simulink model "Model_TranslationEngine64"  (R2022b)
settings: Solver=FixedStepDiscrete  StartTime=0.0  StopTime=5  RelTol=1e-3  EnableMultiTasking=on
InitFcn:
  | % Initialize model
  | ModelSettings=BTConfig.GetModelSettings();
  | 
  | ModelSettings.Validate();
  | 
  | ModelInit;
  | 
  | 
  | % load library data
  | GainLibrary_data;
  | % Load saved values from partition process
  | CapturedConstMask.LoadMapFromFile(bdroot)
StartFcn:
  | % make sure all the simulated RTC requests are found
  | %RTC_SIM_OBJ.ValidateREQs();
undefined symbols (not defined in the file or in its folder): AA, BPLP, Column, NumHFRefBPF, NumHFRefLPF, NumMusicChannels, Row, VolumeMuteConfig
libraries: TuneVar x925, TOP x490, FeaturePath x111, CapturedConstLib x52
(part 31 of 34)

== matlab function Model_TranslationEngine64/NEAR/Near1p1/DrProc/RouterDr/InnerLink/Trivial Translation ==
  data: OutMap output; Map input; nInRouterMask parameter
  events: trigger input FUNCTION_CALL_EVENT
function OutMap  = fcn(Map, nInRouterMask)
%#codegen

% ----- To access TuneVar maximum size, current size, and current value:
%   Note: TuneVar signals arrive with exposed variable size information.
%         The expressions below illustrate for the "Map" input argument.
%
%   size(Map.Value) : the maximum possible size of the Map variable
%
%   Tune.Size   : the current size of *valid* data in Map.Value
%
%   Map.Size(1) : Number of rows present in Map - this does not vary.
%
%   Map.Size(2) : Number of columns currently valid in Map - this is
%       the variable part of size that can change (if allowed by TuneVar).
%
%   Map.Value : the current value of the tune variable... but end-padded 
%       to the maximum available size with undefined/invalid data.
%
%   numel(Map.Value) : another way of looking at the maximum number of
%       elements that could arrive in Map.Value
%
% ----- To register an error, use the following method (works like printf):
%   TranslateError( <format string>, <arguments ... )
%   ... this error will cause the build process to abort.


% The below logic ensures that an output map gets filled in in the 
% "round robin" manner. This is to occur when the supplied map is shorter
% than the number of channel outputs. For instance,
% nChanIn = 4
% nChanOut = 9
% outputMapSupplied = [4 3 2 2]
% 
% This logic would run and return OutMap = [4 3 2 2 1 2 3 4 1]
%
% If no outputMap was supplied (i.e. = [];) THEN
% This logic would run and return OutMap = [1 2 3 4 1 2 3 4 1];


% First part finds the number of output map indices that were left blank
nChanOut = numel(Map.Value);
mapLength = Map.Size(2);
mapDifference = nChanOut - mapLength;
OutMap = int32(Map.Value);

% This loop appropriates the correct input channel number to the
% corresponding output channel, based on the mapDifference found above
if (mapLength == 1) && Map.Value(1) == 0
    mapLength = 0;
    mapDifference = nChanOut;
end
endOfMap = 0;
loopCount = 0;
while endOfMap < mapDifference
    for inputChan = 1 : nInRouterMask
        OutMap(mapLength+inputChan+loopCount) = inputChan;
        endOfMap = endOfMap + 1;
        if endOfMap == mapDifference
            break
        end
    end
    inputChan = 1;
    loopCount = loopCount + nInRouterMask;
end

== matlab function Model_TranslationEngine64/NEAR/Near1p1/DrProc/Upmixer1p1Dr/Subsystem1/Translation ==
  data: mix output single; F1 input; F2 input; F3 input; F4 input; F5 input; F6 input; F7 input; LFI0 input; LFT0 input; RFI0 input; RFT0 input; LSI0 input; LST0 input; RSI0 input; RST0 input; LCI0 input; LCT0 input; RCI0 input; RCT0 input; LFI1 input; LFT1 input; RFI1 input; RFT1 input; LSI1 input; LST1 input; RSI1 input; RST1 input; LCI1 input; LCT1 input; RCI1 input; RCT1 input; nv0l input; nv0r input; nv1l input; nv1r input; FrontPeripheralChannelCount parameter; HeadrestCount parameter; ChannelsPerHeadrest parameter
  events: trigger input FUNCTION_CALL_EVENT
function mix  = fcn(    F1,...
                        F2,...
                        F3,...
                        F4,...
                        F5,...
                        F6,...
                        F7,...
                        LFI0,...
                        LFT0,...
                        RFI0,...
                        RFT0,...
                        LSI0,...
                        LST0,...
                        RSI0,...
                        RST0,...
                        LCI0,...
                        LCT0,...
                        RCI0,...
                        RCT0,...
                        LFI1,...
                        LFT1,...
                        RFI1,...
                        RFT1,...
                        LSI1,...
                        LST1,...
                        RSI1,...
                        RST1,...
                        LCI1,...
                        LCT1,...
                        RCI1,...
                        RCT1,...
                        nv0l,...
                        nv0r,...
                        nv1l,...
                        nv1r, ...
                        FrontPeripheralChannelCount, HeadrestCount, ChannelsPerHeadrest)

% mix = cat(3, F1.Value, F1.Value);                    
% mix = cat(              3,... 
%                         F1.Value,...
%                         F2.Value,...
%                         F3.Value,...
%                         F4.Value,...
%                         F5.Value,...
%                         F6.Value,...
%                         F7.Value,...
%                         LFI0.Value,...
%                         LFT0.Value,...
%                         RFI0.Value,...
%                         RFT0.Value,...
%                         LSI0.Value,...
%                         LST0.Value,...
%                         RSI0.Value,...
%                         RST0.Value,...
%                         LCI0.Value,...
%                         LCT0.Value,...
%                         RCI0.Value,...
%                         RCT0.Value,...
%                         LFI1.Value,...
%                         LFT1.Value,...
%                         RFI1.Value,...
%                         RFT1.Value,...
%                         LSI1.Value,...
%                         LST1.Value,...
%                         RSI1.Value,...
%                         RST1.Value,...
%                         LCI1.Value,...
%                         LCT1.Value,...
%                         RCI1.Value,...
%                         RCT1.Value,...
%                         nv0l.Value,...
%                         nv0r.Value,...
%                         nv1l.Value,...
%                         nv1r.Value);

% f = size(fArr, 1);
% hr = size(hrArr, 1);
% cph = size(cphArr, 1);
f = FrontPeripheralChannelCount;
hr = HeadrestCount;
cph = ChannelsPerHeadrest;
mixSize = f + hr*cph;
% s = size(F1.Value, 1);
s = size(LFI0.Value, 1);
mix = single(zeros(s, s, mixSize));

x = cat(3, F1.Value, F2.Value, F3.Value, F4.Value, F5.Value, F6.Value, F7.Value);
mix(:,:,1:f) = x(:,:,1:f);
if cph == 14
    x = cat(        3,... 
                    LFI0.Value,...
                    LFT0.Value,...
                    RFI0.Value,...
                    RFT0.Value,...
                    LSI0.Value,...
                    LST0.Value,...
                    RSI0.Value,...
                    RST0.Value,...
                    LCI0.Value,...
                    LCT0.Value,...
                    RCI0.Value,...
                    RCT0.Value);
    mix(:,:,f+1:f+12) = x;
	if hr == 2
        x = cat(    3,... 
                    LFI1.Value,...
                    LFT1.Value,...
                    RFI1.Value,...
                    RFT1.Value,...
                    LSI1.Value,...
                    LST1.Value,...
                    RSI1.Value,...
                    RST1.Value,...
                    LCI1.Value,...
                    LCT1.Value,...
                    RCI1.Value,...
                    RCT1.Value);
        mix(:,:,f+13:f+24) = x;
	end
end
x = cat(    3,... 
            nv0l.Value,...
            nv0r.Value);
mix(:,:,f+((cph-2)*hr)+1:f+((cph-2)*hr)+2) = x;
if hr == 2
	x = cat(    3,... 
                nv1l.Value,...
                nv1r.Value);
    mix(:,:,f+((cph-2)*hr)+3:f+((cph-2)*hr)+4) = x;
end
end

== matlab function Model_TranslationEngine64/NEAR/Near1p1/FrProc/Subsystem/FsEQFr/Pooliir/PoolIirTunableWithReset/Translation ==
  data: RawSOS input; NumStages input; PoolNumStages output; PoolCoeffs output; MaxNumStages parameter; VariantUint8 parameter; NumChannels input
  events: trigger input FUNCTION_CALL_EVENT
function [PoolNumStages, PoolCoeffs] = pooliirTranslation(RawSOS, NumStages, MaxNumStages, VariantUint8,  NumChannels)
%#codegen

% Translation from raw SOS for pool SOS

% Some build time sanity size checking before calling the translation
if numel(NumStages.Value) ~= NumChannels
    error('Size of num stages has to match number of input channels')
end

if RawSOS.Size(2) ~= 6
    error ('Coefficient pool matrix must have 6 columns')
end

[PoolNumStages, PoolCoeffs] = poolIirTranslation(RawSOS, NumStages, MaxNumStages, VariantUint8);

% VariantStr = char(VariantUint8);
% switch (VariantStr)
%     case {"Generic","SharcPlusCore"}
%         % These variants order biquad coefficients in a compacted form
%         [PoolNumStages, PoolCoeffs] = pooliirTranslationFcn(RawSOS, NumStages, MaxNumStages);
%     case {"SharcPlusAccelGul","SharcPlusAccelGxp"}
%         % These variants order biquad coefficients for the ADI accelerator
%         [PoolNumStages, PoolCoeffs] = pooliirAccelTranslationFcn(RawSOS, NumStages, MaxNumStages);
%     case{"Hexagon"}
%         % Hexagon specific order for biquad coefficients 
%         [PoolNumStages, PoolCoeffs] = PoolIirHexagonTranslationFcn(RawSOS, NumStages, MaxNumStages);
%     case{"ArmNeonV7V8"}
%         [PoolNumStages, PoolCoeffs] = PoolIirArmNeonV7V8TranslationFcn(RawSOS, NumStages, MaxNumStages);
%     otherwise
%         % This is a build-time error, not a translation error. The
%         % selected build-time variant is not supported for translation
%         error('Invalid implementation type: [%s]', VariantStr);
% end

end

== matlab function Model_TranslationEngine64/NEAR/Near1p1/FrProc/Subsystem/HrEQFr/Subsystem2/Translation ==
  data: eqdelays output single; driversrc1 input; driversrc2 input; driversrc3 input; driversrc4 input; passengersrc1 input; passengersrc2 input; passengersrc3 input; passengersrc4 input; NumHeadrestSpeakers parameter; AnnChannelCount parameter
  events: trigger input FUNCTION_CALL_EVENT
function eqdelays  = fcn(driversrc1, driversrc2, driversrc3, driversrc4, passengersrc1, passengersrc2, passengersrc3, passengersrc4, NumHeadrestSpeakers, AnnChannelCount)
    switch NumHeadrestSpeakers
        case 1
            switch AnnChannelCount
                case 1
                    eqdelays = single([driversrc1.Value, driversrc2.Value]);
                case 2
                    eqdelays = single([driversrc1.Value, driversrc2.Value]);
                case 3
                    eqdelays = single([driversrc1.Value, driversrc2.Value, driversrc3.Value]);
                case 4
                    eqdelays = single([driversrc1.Value, driversrc2.Value, driversrc3.Value, driversrc4.Value]);
            end
        case 2
            switch AnnChannelCount
                case 1
                    eqdelays = single([driversrc1.Value, driversrc2.Value, passengersrc1.Value, passengersrc2.Value]);
                case 2
                    eqdelays = single([driversrc1.Value, driversrc2.Value, passengersrc1.Value, passengersrc2.Value]);
                case 3
                    eqdelays = single([driversrc1.Value, driversrc2.Value, driversrc3.Value, passengersrc1.Value, passengersrc2.Value, passengersrc3.Value]);
                case 4
                    eqdelays = single([driversrc1.Value, driversrc2.Value, driversrc3.Value, driversrc4.Value, passengersrc1.Value, passengersrc2.Value, passengersrc3.Value, passengersrc4.Value]);
            end
    end

end

== matlab function Model_TranslationEngine64/NEAR/Near1p1/FrProc/Subsystem/HrEQFr/PoolIirTunable/PoolIirTunableWithReset/Translation ==
  data: RawSOS input; NumStages input; PoolNumStages output; PoolCoeffs output; MaxNumStages parameter; VariantUint8 parameter; NumChannels input
  events: trigger input FUNCTION_CALL_EVENT
function [PoolNumStages, PoolCoeffs] = pooliirTranslation(RawSOS, NumStages, MaxNumStages, VariantUint8,  NumChannels)
%#codegen

% Translation from raw SOS for pool SOS

% Some build time sanity size checking before calling the translation
if numel(NumStages.Value) ~= NumChannels
    error('Size of num stages has to match number of input channels')
end

if RawSOS.Size(2) ~= 6
    error ('Coefficient pool matrix must have 6 columns')
end

[PoolNumStages, PoolCoeffs] = poolIirTranslation(RawSOS, NumStages, MaxNumStages, VariantUint8);

% VariantStr = char(VariantUint8);
% switch (VariantStr)
%     case {"Generic","SharcPlusCore"}
%         % These variants order biquad coefficients in a compacted form
%         [PoolNumStages, PoolCoeffs] = pooliirTranslationFcn(RawSOS, NumStages, MaxNumStages);
%     case {"SharcPlusAccelGul","SharcPlusAccelGxp"}
%         % These variants order biquad coefficients for the ADI accelerator
%         [PoolNumStages, PoolCoeffs] = pooliirAccelTranslationFcn(RawSOS, NumStages, MaxNumStages);
%     case{"Hexagon"}
%         % Hexagon specific order for biquad coefficients 
%         [PoolNumStages, PoolCoeffs] = PoolIirHexagonTranslationFcn(RawSOS, NumStages, MaxNumStages);
%     case{"ArmNeonV7V8"}
%         [PoolNumStages, PoolCoeffs] = PoolIirArmNeonV7V8TranslationFcn(RawSOS, NumStages, MaxNumStages);
%     otherwise
%         % This is a build-time error, not a translation error. The
%         % selected build-time variant is not supported for translation
%         error('Invalid implementation type: [%s]', VariantStr);
% end

end

== matlab function Model_TranslationEngine64/NEAR/Near1p1/VolumeMute/AnnouncementLevelDetector/ch2_level/hold_time/sec2samples ==
  data: y output; u input; FrameRate parameter
  events: trigger input FUNCTION_CALL_EVENT
function y  = fcn(u,FrameRate)
%#codegen

y = ceil(u.Value*FrameRate);

== matlab function Model_TranslationEngine64/ModelPreAmp/DecRate/AudioPilot35/Audiopilot_3_5/GainApplication/Compensation/MidrangeLpf/LinkwitzRiley ==
  data: num output; freq input; denom output; SampleRate parameter
  events: trigger input FUNCTION_CALL_EVENT
function [num,denom] = fcn(freq,SampleRate)
% Forms the numerator and denominator coefficients
% for a 4th order Linkwitz-Riley low-pass filter with 
% the specified cutoff frequency 
%#codegen

Fc = freq.Value;
FiltOrder = 4;  % This is hard-coded

[Z,P,K] = LinkwitzRileyFiltDesign(FiltOrder,Fc/(SampleRate/2),'low');
[num, denom] = zp2tf(Z,P,K);

== matlab function Model_TranslationEngine64/NEAR/Near1p1/FrProc/Subsystem/RouterFr/InnerLink/Trivial Translation ==
  data: OutMap output; Map input; nInRouterMask parameter
  events: trigger input FUNCTION_CALL_EVENT
function OutMap  = fcn(Map, nInRouterMask)
%#codegen

% ----- To access TuneVar maximum size, current size, and current value:
%   Note: TuneVar signals arrive with exposed variable size information.
%         The expressions below illustrate for the "Map" input argument.
%
%   size(Map.Value) : the maximum possible size of the Map variable
%
%   Tune.Size   : the current size of *valid* data in Map.Value
%
%   Map.Size(1) : Number of rows present in Map - this does not vary.
%
%   Map.Size(2) : Number of columns currently valid in Map - this is
%       the variable part of size that can change (if allowed by TuneVar).
%
%   Map.Value : the current value of the tune variable... but end-padded 
%       to the maximum available size with undefined/invalid data.
%
%   numel(Map.Value) : another way of looking at the maximum number of
%       elements that could arrive in Map.Value
%
% ----- To register an error, use the following method (works like printf):
%   TranslateError( <format string>, <arguments ... )
%   ... this error will cause the build process to abort.


% The below logic ensures that an output map gets filled in in the 
% "round robin" manner. This is to occur when the supplied map is shorter
% than the number of channel outputs. For instance,
% nChanIn = 4
% nChanOut = 9
% outputMapSupplied = [4 3 2 2]
% 
% This logic would run and return OutMap = [4 3 2 2 1 2 3 4 1]
%
% If no outputMap was supplied (i.e. = [];) THEN
% This logic would run and return OutMap = [1 2 3 4 1 2 3 4 1];


% First part finds the number of output map indices that were left blank
nChanOut = numel(Map.Value);
mapLength = Map.Size(2);
mapDifference = nChanOut - mapLength;
OutMap = int32(Map.Value);

% This loop appropriates the correct input channel number to the
% corresponding output channel, based on the mapDifference found above
if (mapLength == 1) && Map.Value(1) == 0
    mapLength = 0;
    mapDifference = nChanOut;
end
endOfMap = 0;
loopCount = 0;
while endOfMap < mapDifference
    for inputChan = 1 : nInRouterMask
        OutMap(mapLength+inputChan+loopCount) = inputChan;
        endOfMap = endOfMap + 1;
        if endOfMap == mapDifference
            break
        end
    end
    inputChan = 1;
    loopCount = loopCount + nInRouterMask;
end

== matlab function Model_TranslationEngine64/NEAR/Near1p1/FrProc/Subsystem/Upmixer1p1Fr/Subsystem1/Translation ==
  data: mix output single; F1 input; F2 input; F3 input; F4 input; F5 input; F6 input; F7 input; LFI0 input; LFT0 input; RFI0 input; RFT0 input; LSI0 input; LST0 input; RSI0 input; RST0 input; LCI0 input; LCT0 input; RCI0 input; RCT0 input; LFI1 input; LFT1 input; RFI1 input; RFT1 input; LSI1 input; LST1 input; RSI1 input; RST1 input; LCI1 input; LCT1 input; RCI1 input; RCT1 input; nv0l input; nv0r input; nv1l input; nv1r input; FrontPeripheralChannelCount parameter; HeadrestCount parameter; ChannelsPerHeadrest parameter
  events: trigger input FUNCTION_CALL_EVENT
function mix  = fcn(    F1,...
                        F2,...
                        F3,...
                        F4,...
                        F5,...
                        F6,...
                        F7,...
                        LFI0,...
                        LFT0,...
                        RFI0,...
                        RFT0,...
                        LSI0,...
                        LST0,...
                        RSI0,...
                        RST0,...
                        LCI0,...
                        LCT0,...
                        RCI0,...
                        RCT0,...
                        LFI1,...
                        LFT1,...
                        RFI1,...
                        RFT1,...
                        LSI1,...
                        LST1,...
                        RSI1,...
                        RST1,...
                        LCI1,...
                        LCT1,...
                        RCI1,...
                        RCT1,...
                        nv0l,...
                        nv0r,...
                        nv1l,...
                        nv1r, ...
                        FrontPeripheralChannelCount, HeadrestCount, ChannelsPerHeadrest)

% mix = cat(3, F1.Value, F1.Value);                    
% mix = cat(              3,... 
%                         F1.Value,...
%                         F2.Value,...
%                         F3.Value,...
%                         F4.Value,...
%                         F5.Value,...
%                         F6.Value,...
%                         F7.Value,...
%                         LFI0.Value,...
%                         LFT0.Value,...
%                         RFI0.Value,...
%                         RFT0.Value,...
%                         LSI0.Value,...
%                         LST0.Value,...
%                         RSI0.Value,...
%                         RST0.Value,...
%                         LCI0.Value,...
%                         LCT0.Value,...
%                         RCI0.Value,...
%                         RCT0.Value,...
%                         LFI1.Value,...
%                         LFT1.Value,...
%                         RFI1.Value,...
%                         RFT1.Value,...
%                         LSI1.Value,...
%                         LST1.Value,...
%                         RSI1.Value,...
%                         RST1.Value,...
%                         LCI1.Value,...
%                         LCT1.Value,...
%                         RCI1.Value,...
%                         RCT1.Value,...
%                         nv0l.Value,...
%                         nv0r.Value,...
%                         nv1l.Value,...
%                         nv1r.Value);

% f = size(fArr, 1);
% hr = size(hrArr, 1);
% cph = size(cphArr, 1);
f = FrontPeripheralChannelCount;
hr = HeadrestCount;
cph = ChannelsPerHeadrest;
mixSize = f + hr*cph;
% s = size(F1.Value, 1);
s = size(LFI0.Value, 1);
mix = single(zeros(s, s, mixSize));

x = cat(3, F1.Value, F2.Value, F3.Value, F4.Value, F5.Value, F6.Value, F7.Value);
mix(:,:,1:f) = x(:,:,1:f);
if cph == 14
    x = cat(        3,... 
                    LFI0.Value,...
                    LFT0.Value,...
                    RFI0.Value,...
                    RFT0.Value,...
                    LSI0.Value,...
                    LST0.Value,...
                    RSI0.Value,...
                    RST0.Value,...
                    LCI0.Value,...
                    LCT0.Value,...
                    RCI0.Value,...
                    RCT0.Value);
    mix(:,:,f+1:f+12) = x;
	if hr == 2
        x = cat(    3,... 
                    LFI1.Value,...
                    LFT1.Value,...
                    RFI1.Value,...
                    RFT1.Value,...
                    LSI1.Value,...
                    LST1.Value,...
                    RSI1.Value,...
                    RST1.Value,...
                    LCI1.Value,...
                    LCT1.Value,...
                    RCI1.Value,...
                    RCT1.Value);
        mix(:,:,f+13:f+24) = x;
	end
end
x = cat(    3,... 
            nv0l.Value,...
            nv0r.Value);
mix(:,:,f+((cph-2)*hr)+1:f+((cph-2)*hr)+2) = x;
if hr == 2
	x = cat(    3,... 
                nv1l.Value,...
                nv1r.Value);
    mix(:,:,f+((cph-2)*hr)+3:f+((cph-2)*hr)+4) = x;
end
end

== matlab function Model_TranslationEngine64/NEAR/Near1p1/VolumeMute/AnnouncementLevelDetector/ch2_level/slow_decay/sec2samples ==
  data: y output; u input; FrameRate parameter
  events: trigger input FUNCTION_CALL_EVENT
function y  = fcn(u,FrameRate)
%#codegen

y = -abs(u.Value/FrameRate);

== matlab function Model_TranslationEngine64/NEAR/Near1p1/VolumeMute/AnnouncementLevelDetector/ch3_level/fast_decay/sec2samples ==
  data: y output; u input; FrameRate parameter
  events: trigger input FUNCTION_CALL_EVENT
function y  = fcn(u,FrameRate)
%#codegen

y = -abs(u.Value/FrameRate);

== matlab function Model_TranslationEngine64/NEAR/Near1p1/VolumeMute/AnnouncementLevelDetector/ch3_level/hold_margin/SetPositive ==
  data: TOP output single; Tune input
  events: trigger input FUNCTION_CALL_EVENT
function TOP = fcn(Tune)
%#codegen

TOP = abs(Tune.Value);

== matlab function Model_TranslationEngine64/NEAR/Near1p1/VolumeMute/AnnouncementLevelDetector/ch3_level/hold_time/sec2samples ==
  data: y output; u input; FrameRate parameter
  events: trigger input FUNCTION_CALL_EVENT
function y  = fcn(u,FrameRate)
%#codegen

y = ceil(u.Value*FrameRate);

== matlab function Model_TranslationEngine64/NEAR/Near1p1/VolumeMute/AnnouncementLevelDetector/ch3_level/slow_decay/sec2samples ==
  data: y output; u input; FrameRate parameter
  events: trigger input FUNCTION_CALL_EVENT
function y  = fcn(u,FrameRate)
%#codegen

y = -abs(u.Value/FrameRate);

== matlab function Model_TranslationEngine64/ModelPreAmp/DecRate/AudioPilot35/Audiopilot_3_5/NoiseEstimationVariant/RegularNoiseEstimation/HFNoiseEstimatorCoh/PreProcessing/Anti-Aliasing Filter/InnerLink/PoolIirTunableWithReset/Translation ==
  data: RawSOS input; NumStages input; PoolNumStages output; PoolCoeffs output; MaxNumStages parameter; VariantUint8 parameter; NumChannels input
  events: trigger input FUNCTION_CALL_EVENT
function [PoolNumStages, PoolCoeffs] = pooliirTranslation(RawSOS, NumStages, MaxNumStages, VariantUint8,  NumChannels)
%#codegen

% Translation from raw SOS for pool SOS

% Some build time sanity size checking before calling the translation
if numel(NumStages.Value) ~= NumChannels
    error('Size of num stages has to match number of input channels')
end

if RawSOS.Size(2) ~= 6
    error ('Coefficient pool matrix must have 6 columns')
end

[PoolNumStages, PoolCoeffs] = poolIirTranslation(RawSOS, NumStages, MaxNumStages, VariantUint8);

% VariantStr = char(VariantUint8);
% switch (VariantStr)
%     case {"Generic","SharcPlusCore"}
%         % These variants order biquad coefficients in a compacted form
%         [PoolNumStages, PoolCoeffs] = pooliirTranslationFcn(RawSOS, NumStages, MaxNumStages);
%     case {"SharcPlusAccelGul","SharcPlusAccelGxp"}
%         % These variants order biquad coefficients for the ADI accelerator
%         [PoolNumStages, PoolCoeffs] = pooliirAccelTranslationFcn(RawSOS, NumStages, MaxNumStages);
%     case{"Hexagon"}
%         % Hexagon specific order for biquad coefficients 
%         [PoolNumStages, PoolCoeffs] = PoolIirHexagonTranslationFcn(RawSOS, NumStages, MaxNumStages);
%     case{"ArmNeonV7V8"}
%         [PoolNumStages, PoolCoeffs] = PoolIirArmNeonV7V8TranslationFcn(RawSOS, NumStages, MaxNumStages);
%     otherwise
%         % This is a build-time error, not a translation error. The
%         % selected build-time variant is not supported for translation
%         error('Invalid implementation type: [%s]', VariantStr);
% end

end

== matlab function Model_TranslationEngine64/NEAR/Near1p1/VolumeMute/AnnouncementLevelDetector/ch4_level/fast_decay/sec2samples ==
  data: y output; u input; FrameRate parameter
  events: trigger input FUNCTION_CALL_EVENT
function y  = fcn(u,FrameRate)
%#codegen

y = -abs(u.Value/FrameRate);

== matlab function Model_TranslationEngine64/NEAR/Near1p1/VolumeMute/AnnouncementLevelDetector/ch4_level/hold_margin/SetPositive ==
  data: TOP output single; Tune input
  events: trigger input FUNCTION_CALL_EVENT
function TOP = fcn(Tune)
%#codegen

TOP = abs(Tune.Value);

== matlab function Model_TranslationEngine64/NEAR/Near1p1/VolumeMute/AnnouncementLevelDetector/ch4_level/hold_time/sec2samples ==
  data: y output; u input; FrameRate parameter
  events: trigger input FUNCTION_CALL_EVENT
function y  = fcn(u,FrameRate)
%#codegen

y = ceil(u.Value*FrameRate);

== matlab function Model_TranslationEngine64/NEAR/Near1p1/VolumeMute/AnnouncementLevelDetector/ch4_level/slow_decay/sec2samples ==
  data: y output; u input; FrameRate parameter
  events: trigger input FUNCTION_CALL_EVENT
function y  = fcn(u,FrameRate)
%#codegen

y = -abs(u.Value/FrameRate);

== matlab function Model_TranslationEngine64/NEAR/Near1p1/VolumeMute/VolMuteCh1/Ann1NonEntGainCalc/TuneTOP8/translation ==
  data: Num output size=[1,2]; tau input size=1; Den output size=[1,2]; Fd parameter
  events: trigger input FUNCTION_CALL_EVENT
function [Num, Den]  = fcn(tau, Fd)
%
% Calculate coefficients for single pole LPF
%

Wc      = 1/(tau.Value*Fd);
sinCoef = sin(Wc);
cosCoef = cos(Wc);
coef    = (1-sinCoef)/cosCoef;

Num = double([1-coef 0]);
Den =  double([1 -(coef)]);

== matlab function Model_TranslationEngine64/NEAR/Near1p1/VolumeMute/AnnouncementLevelDetector/PreProcessing/PreEmphasisShelfFilter/PoolIirTunableWithReset/Translation ==
  data: RawSOS input; NumStages input; PoolNumStages output; PoolCoeffs output; MaxNumStages parameter; VariantUint8 parameter; NumChannels input
  events: trigger input FUNCTION_CALL_EVENT
function [PoolNumStages, PoolCoeffs] = pooliirTranslation(RawSOS, NumStages, MaxNumStages, VariantUint8,  NumChannels)
%#codegen

% Translation from raw SOS for pool SOS

% Some build time sanity size checking before calling the translation
if numel(NumStages.Value) ~= NumChannels
    error('Size of num stages has to match number of input channels')
end

if RawSOS.Size(2) ~= 6
    error ('Coefficient pool matrix must have 6 columns')
end

[PoolNumStages, PoolCoeffs] = poolIirTranslation(RawSOS, NumStages, MaxNumStages, VariantUint8);

% VariantStr = char(VariantUint8);
% switch (VariantStr)
%     case {"Generic","SharcPlusCore"}
%         % These variants order biquad coefficients in a compacted form
%         [PoolNumStages, PoolCoeffs] = pooliirTranslationFcn(RawSOS, NumStages, MaxNumStages);
%     case {"SharcPlusAccelGul","SharcPlusAccelGxp"}
%         % These variants order biquad coefficients for the ADI accelerator
%         [PoolNumStages, PoolCoeffs] = pooliirAccelTranslationFcn(RawSOS, NumStages, MaxNumStages);
%     case{"Hexagon"}
%         % Hexagon specific order for biquad coefficients 
%         [PoolNumStages, PoolCoeffs] = PoolIirHexagonTranslationFcn(RawSOS, NumStages, MaxNumStages);
%     case{"ArmNeonV7V8"}
%         [PoolNumStages, PoolCoeffs] = PoolIirArmNeonV7V8TranslationFcn(RawSOS, NumStages, MaxNumStages);
%     otherwise
%         % This is a build-time error, not a translation error. The
%         % selected build-time variant is not supported for translation
%         error('Invalid implementation type: [%s]', VariantStr);
% end

end

== matlab function Model_TranslationEngine64/NEAR/Near1p1/VolumeMute/VolMuteCh2/Ann2NonEntVncApplied/nonentVNCApplied_subsystem/TuneTOP/Translation ==
  data: Num output; tau input; Fs input; L input; Den output
  events: trigger input FUNCTION_CALL_EVENT
function [Num, Den]  = fcn(tau, Fs, L)

f0 = 1/tau.Value;   % Approximation of cutoff freq from lpf filter time constant

fs_lpf = Fs/L;        % lpf filtter sample rate

% [Num, Den]= butter(1,2*f0/fs_lpf);  % butter() doesn't work with dynamic parameters
[Num, Den] = firstOrderButter(fs_lpf,f0);  % Calculation of lpf filter coefficients

== matlab function Model_TranslationEngine64/NEAR/Near1p1/VolumeMute/VolMuteCh2/Ann2NonEntGainCalc/TuneTOP8/translation ==
  data: Num output size=[1,2]; tau input size=1; Den output size=[1,2]; Fd parameter
  events: trigger input FUNCTION_CALL_EVENT
function [Num, Den]  = fcn(tau, Fd)
%
% Calculate coefficients for single pole LPF
%

Wc      = 1/(tau.Value*Fd);
sinCoef = sin(Wc);
cosCoef = cos(Wc);
coef    = (1-sinCoef)/cosCoef;

Num = double([1-coef 0]);
Den =  double([1 -(coef)]);

== matlab function Model_TranslationEngine64/NEAR/Near1p1/VolumeMute/VolMuteCh3/Ann3NonEntVncApplied/nonentVNCApplied_subsystem/TuneTOP/Translation ==
  data: Num output; tau input; Fs input; L input; Den output
  events: trigger input FUNCTION_CALL_EVENT
function [Num, Den]  = fcn(tau, Fs, L)

f0 = 1/tau.Value;   % Approximation of cutoff freq from lpf filter time constant

fs_lpf = Fs/L;        % lpf filtter sample rate

% [Num, Den]= butter(1,2*f0/fs_lpf);  % butter() doesn't work with dynamic parameters
[Num, Den] = firstOrderButter(fs_lpf,f0);  % Calculation of lpf filter coefficients

== matlab function Model_TranslationEngine64/NEAR/Near1p1/VolumeMute/VolMuteCh3/Ann3NonEntGainCalc/TuneTOP8/translation ==
  data: Num output size=[1,2]; tau input size=1; Den output size=[1,2]; Fd parameter
  events: trigger input FUNCTION_CALL_EVENT
function [Num, Den]  = fcn(tau, Fd)
%
% Calculate coefficients for single pole LPF
%

Wc      = 1/(tau.Value*Fd);
sinCoef = sin(Wc);
cosCoef = cos(Wc);
coef    = (1-sinCoef)/cosCoef;

Num = double([1-coef 0]);
Den =  double([1 -(coef)]);

== matlab function Model_TranslationEngine64/NEAR/Near1p1/VolumeMute/VolMuteCh4/Ann4NonEntVncApplied/nonentVNCApplied_subsystem/TuneTOP/Translation ==
  data: Num output; tau input; Fs input; L input; Den output
  events: trigger input FUNCTION_CALL_EVENT
function [Num, Den]  = fcn(tau, Fs, L)

f0 = 1/tau.Value;   % Approximation of cutoff freq from lpf filter time constant

fs_lpf = Fs/L;        % lpf filtter sample rate

% [Num, Den]= butter(1,2*f0/fs_lpf);  % butter() doesn't work with dynamic parameters
[Num, Den] = firstOrderButter(fs_lpf,f0);  % Calculation of lpf filter coefficients

== matlab function Model_TranslationEngine64/NEAR/Near1p1/VolumeMute/VolMuteCh1/Volume/volume table translation ==
  data: Table_Idx output; Table_dB output; VolumeTable input
  events: trigger input FUNCTION_CALL_EVENT
function [Table_Idx,Table_dB] = fcn(VolumeTable)
%#codegen
%
% Demux Volume Table matrix into an index vector amd gain vector
%

% Set up the size and datatype of our TOP outputs:
maxTableSize = numel(VolumeTable.Value) / 2;
idxType = 'uint8';
idxStorageType = 'uint32';
dbType = 'single';
Table_Idx = zeros(1,maxTableSize,idxStorageType);
Table_dB = zeros(1,maxTableSize,dbType);

% separate the pairs into their index and value components
givenPairs = VolumeTable.Size(1);
indexes = VolumeTable.Value(1:givenPairs,1);
values = VolumeTable.Value(1:givenPairs,2);

% then sort and ignore duplicates
[cleanIdx,map] = unique(indexes);

% Validate input sizes
numPairs = numel(map);
argName='VolumeTable';

% Validate: enough data?
if (numPairs < 2)
    TranslateError('%s must have at least 2 index pairs. Encounted value with only %f pairs\n', argName, numPairs);
end

% Validate: Highest index still below 1.0?
if (cleanIdx(end) > 1)
    TranslateError('%s out of range table index %f encountered. Index must be between 0 and 1.\n',argName,cleanIdx(end));
end

% fill in the table buffer with provided pairs
for i=1:numPairs
    Table_Idx(i) = intmax(idxType) * cleanIdx(i);
    Table_dB(i) = values(map(i));
end
% fill the rest of the table buffer with the last entry
for j=numel(map)+1:maxTableSize
    Table_Idx(j) = Table_Idx(numPairs);
    Table_dB(j) =  Table_dB(numPairs);
end

end

== matlab function Model_TranslationEngine64/NEAR/Near1p1/VolumeMute/VolMuteCh4/Ann4NonEntGainCalc/TuneTOP8/translation ==
  data: Num output size=[1,2]; tau input size=1; Den output size=[1,2]; Fd parameter
  events: trigger input FUNCTION_CALL_EVENT
function [Num, Den]  = fcn(tau, Fd)
%
% Calculate coefficients for single pole LPF
%

Wc      = 1/(tau.Value*Fd);
sinCoef = sin(Wc);
cosCoef = cos(Wc);
coef    = (1-sinCoef)/cosCoef;

Num = double([1-coef 0]);
Den =  double([1 -(coef)]);

== matlab function Model_TranslationEngine64/ModelPreAmp/DecRate/AudioPilot35/Audiopilot_3_5/GainCalculation/BoostMapAdjustment/AudiopilotOn/Bass0Enable ==
  data: on input; slopeOut output; slope input
  events: trigger input FUNCTION_CALL_EVENT
function slopeOut  = enable(on,slope)
%#codegen
slopeOut = slope.Value * on.Value;

== matlab function Model_TranslationEngine64/PostProcess/PostProcess/PostLimiterEQ/PoolIirTunableWithReset/Translation ==
  data: RawSOS input; NumStages input; PoolNumStages output; PoolCoeffs output; MaxNumStages parameter; VariantUint8 parameter; NumChannels input
  events: trigger input FUNCTION_CALL_EVENT
function [PoolNumStages, PoolCoeffs] = pooliirTranslation(RawSOS, NumStages, MaxNumStages, VariantUint8,  NumChannels)
%#codegen

% Translation from raw SOS for pool SOS

% Some build time sanity size checking before calling the translation
if numel(NumStages.Value) ~= NumChannels
    error('Size of num stages has to match number of input channels')
end

if RawSOS.Size(2) ~= 6
    error ('Coefficient pool matrix must have 6 columns')
end

[PoolNumStages, PoolCoeffs] = poolIirTranslation(RawSOS, NumStages, MaxNumStages, VariantUint8);

% VariantStr = char(VariantUint8);
% switch (VariantStr)
%     case {"Generic","SharcPlusCore"}
%         % These variants order biquad coefficients in a compacted form
%         [PoolNumStages, PoolCoeffs] = pooliirTranslationFcn(RawSOS, NumStages, MaxNumStages);
%     case {"SharcPlusAccelGul","SharcPlusAccelGxp"}
%         % These variants order biquad coefficients for the ADI accelerator
%         [PoolNumStages, PoolCoeffs] = pooliirAccelTranslationFcn(RawSOS, NumStages, MaxNumStages);
%     case{"Hexagon"}
%         % Hexagon specific order for biquad coefficients 
%         [PoolNumStages, PoolCoeffs] = PoolIirHexagonTranslationFcn(RawSOS, NumStages, MaxNumStages);
%     case{"ArmNeonV7V8"}
%         [PoolNumStages, PoolCoeffs] = PoolIirArmNeonV7V8TranslationFcn(RawSOS, NumStages, MaxNumStages);
%     otherwise
%         % This is a build-time error, not a translation error. The
%         % selected build-time variant is not supported for translation
%         error('Invalid implementation type: [%s]', VariantStr);
% end

end

== matlab function Model_TranslationEngine64/NEAR/Near1p1/VolumeMute/VolMuteCh2/Volume/volume table translation ==
  data: Table_Idx output; Table_dB output; VolumeTable input
  events: trigger input FUNCTION_CALL_EVENT
function [Table_Idx,Table_dB] = fcn(VolumeTable)
%#codegen
%
% Demux Volume Table matrix into an index vector amd gain vector
%

% Set up the size and datatype of our TOP outputs:
maxTableSize = numel(VolumeTable.Value) / 2;
idxType = 'uint8';
idxStorageType = 'uint32';
dbType = 'single';
Table_Idx = zeros(1,maxTableSize,idxStorageType);
Table_dB = zeros(1,maxTableSize,dbType);

% separate the pairs into their index and value components
givenPairs = VolumeTable.Size(1);
indexes = VolumeTable.Value(1:givenPairs,1);
values = VolumeTable.Value(1:givenPairs,2);

% then sort and ignore duplicates
[cleanIdx,map] = unique(indexes);

% Validate input sizes
numPairs = numel(map);
argName='VolumeTable';

% Validate: enough data?
if (numPairs < 2)
    TranslateError('%s must have at least 2 index pairs. Encounted value with only %f pairs\n', argName, numPairs);
end

% Validate: Highest index still below 1.0?
if (cleanIdx(end) > 1)
    TranslateError('%s out of range table index %f encountered. Index must be between 0 and 1.\n',argName,cleanIdx(end));
end

% fill in the table buffer with provided pairs
for i=1:numPairs
    Table_Idx(i) = intmax(idxType) * cleanIdx(i);
    Table_dB(i) = values(map(i));
end
% fill the rest of the table buffer with the last entry
for j=numel(map)+1:maxTableSize
    Table_Idx(j) = Table_Idx(numPairs);
    Table_dB(j) =  Table_dB(numPairs);
end

end

== matlab function Model_TranslationEngine64/PostProcess/PostProcess/Limiter/Limiter/MATLAB Function1 ==
  data: u input; y output; Fs input
  events: trigger input FUNCTION_CALL_EVENT
function y = fcn(u, Fs)

% Convert from dB to linear
y = single(undb20(abs(u.Value) / Fs));

== matlab function Model_TranslationEngine64/PostProcess/PostProcess/Limiter/Limiter/MATLAB Function2 ==
  data: u input; y output; Fs input
  events: trigger input FUNCTION_CALL_EVENT
function y = fcn(u, Fs)

% Convert decay value from dB to linear
y = single(undb20(abs(u.Value) / Fs));

== matlab function Model_TranslationEngine64/NEAR/Near1p1/VolumeMute/VolMuteCh3/Volume/volume table translation ==
  data: Table_Idx output; Table_dB output; VolumeTable input
  events: trigger input FUNCTION_CALL_EVENT
function [Table_Idx,Table_dB] = fcn(VolumeTable)
%#codegen
%
% Demux Volume Table matrix into an index vector amd gain vector
%

% Set up the size and datatype of our TOP outputs:
maxTableSize = numel(VolumeTable.Value) / 2;
idxType = 'uint8';
idxStorageType = 'uint32';
dbType = 'single';
Table_Idx = zeros(1,maxTableSize,idxStorageType);
Table_dB = zeros(1,maxTableSize,dbType);

% separate the pairs into their index and value components
givenPairs = VolumeTable.Size(1);
indexes = VolumeTable.Value(1:givenPairs,1);
values = VolumeTable.Value(1:givenPairs,2);

% then sort and ignore duplicates
[cleanIdx,map] = unique(indexes);

% Validate input sizes
numPairs = numel(map);
argName='VolumeTable';

% Validate: enough data?
if (numPairs < 2)
    TranslateError('%s must have at least 2 index pairs. Encounted value with only %f pairs\n', argName, numPairs);
end

% Validate: Highest index still below 1.0?
if (cleanIdx(end) > 1)
    TranslateError('%s out of range table index %f encountered. Index must be between 0 and 1.\n',argName,cleanIdx(end));
end

% fill in the table buffer with provided pairs
for i=1:numPairs
    Table_Idx(i) = intmax(idxType) * cleanIdx(i);
    Table_dB(i) = values(map(i));
end
% fill the rest of the table buffer with the last entry
for j=numel(map)+1:maxTableSize
    Table_Idx(j) = Table_Idx(numPairs);
    Table_dB(j) =  Table_dB(numPairs);
end

end

== matlab function Model_TranslationEngine64/PostProcess/PostProcess/Limiter/Limiter/MATLAB Function3 ==
  data: attackDB input; threshold input; Fs input; attack output; k1 output
  events: trigger input FUNCTION_CALL_EVENT
function [attack, k1]= fcn(attackDB, threshold, Fs)

% This function translates threshold and attackDB into a k1 value
% k1 is used later in the main Limiter function to apply gain redux

% If we find that any channel has a threshold value of zero,
% reset it to 100, for we essentially do not want to limit 
% that specific channel.
minThreshold = 0.001;   % check against small number, set to zero if so. 
threshold.Value(threshold.Value < minThreshold) = 0;
if ~(all(threshold.Value))
    threshold.Value(find(threshold.Value == 0)) = 100;
end

% If we find attack value is 0, set to 10000
if ~(all(attackDB.Value))
    attackDB.Value(find(attackDB.Value == 0)) = 10000;
end

% Set output values
attack = single(1 - undb20(-abs(attackDB.Value) / Fs));
k1 = attack ./ single(threshold.Value);

== matlab function Model_TranslationEngine64/PostProcess/PostProcess/Limiter/Limiter/MATLAB Function4 ==
  data: u input; y output
  events: trigger input FUNCTION_CALL_EVENT
function y = fcn(u)

% Translate from dB to linear
y = single(undb20(-abs(u.Value)));

== matlab function Model_TranslationEngine64/NEAR/Near1p1/VolumeMute/VolMuteCh4/Volume/volume table translation ==
  data: Table_Idx output; Table_dB output; VolumeTable input
  events: trigger input FUNCTION_CALL_EVENT
function [Table_Idx,Table_dB] = fcn(VolumeTable)
%#codegen
%
% Demux Volume Table matrix into an index vector amd gain vector
%

% Set up the size and datatype of our TOP outputs:
maxTableSize = numel(VolumeTable.Value) / 2;
idxType = 'uint8';
idxStorageType = 'uint32';
dbType = 'single';
Table_Idx = zeros(1,maxTableSize,idxStorageType);
Table_dB = zeros(1,maxTableSize,dbType);

% separate the pairs into their index and value components
givenPairs = VolumeTable.Size(1);
indexes = VolumeTable.Value(1:givenPairs,1);
values = VolumeTable.Value(1:givenPairs,2);

% then sort and ignore duplicates
[cleanIdx,map] = unique(indexes);

% Validate input sizes
numPairs = numel(map);
argName='VolumeTable';

% Validate: enough data?
if (numPairs < 2)
    TranslateError('%s must have at least 2 index pairs. Encounted value with only %f pairs\n', argName, numPairs);
end

% Validate: Highest index still below 1.0?
if (cleanIdx(end) > 1)
    TranslateError('%s out of range table index %f encountered. Index must be between 0 and 1.\n',argName,cleanIdx(end));
end

% fill in the table buffer with provided pairs
for i=1:numPairs
    Table_Idx(i) = intmax(idxType) * cleanIdx(i);
    Table_dB(i) = values(map(i));
end
% fill the rest of the table buffer with the last entry
for j=numel(map)+1:maxTableSize
    Table_Idx(j) = Table_Idx(numPairs);
    Table_dB(j) =  Table_dB(numPairs);
end

end

== matlab function Model_TranslationEngine64/PostProcess/PostProcess/Limiter/Limiter/MATLAB Function5 ==
  data: attackDB input; threshold input; Fs input; attack output; k1 output
  events: trigger input FUNCTION_CALL_EVENT
function [attack, k1]= fcn(attackDB, threshold, Fs)

% This function translates threshold and attackDB into a k1 value
% k1 is used later in the main Limiter function to apply gain redux

% If we find that any channel has a threshold value of zero,
% reset it to 100, for we essentially do not want to limit 
% that specific channel.
minThreshold = 0.001;   % check against small number, set to zero if so. 
threshold.Value(threshold.Value < minThreshold) = 0;
if ~(all(threshold.Value))
    threshold.Value(find(threshold.Value == 0)) = 100;
end

% If we find attack value is 0, set to 10000
if ~(all(attackDB.Value))
    attackDB.Value(find(attackDB.Value == 0)) = 10000;
end

% Set output values
attack = single(1 - undb20(-abs(attackDB.Value) / Fs));
k1 = attack ./ single(threshold.Value);

== matlab function Model_TranslationEngine64/PostProcess/PostProcess/Limiter/Limiter/MATLAB Function6 ==
  data: u input; y output
  events: trigger input FUNCTION_CALL_EVENT
function y = fcn(u)

% Convert from dB to linear
y = single(undb20(-abs(u.Value)));

== matlab function Model_TranslationEngine64/ModelPreAmp/DecRate/AudioPilot35/Audiopilot_3_5/GainCalculation/BoostMapAdjustment/AudiopilotOn/Midrange0Enable ==
  data: on input; slopeOut output; slope input
  events: trigger input FUNCTION_CALL_EVENT
function slopeOut  = enable(on,slope)
%#codegen
slopeOut = slope.Value * on.Value;

== matlab function Model_TranslationEngine64/PostProcess/PostProcess/Soft Clipper/SoftClipper/translation ==
  data: ymax_tune input; xmin_top output; xmin_tune input; xmax_top output; p2 output
  events: trigger input FUNCTION_CALL_EVENT
function [xmin_top,xmax_top, p2] = fcn(ymax_tune, xmin_tune)

% Translates Ymax and Xmin to Xmax and Xmin

xmin_top = xmin_tune.Value;
xmax_top = 2 * ymax_tune.Value - xmin_top;

% p2 remains 0 unless below condition is met
% p2 is later used in the gain redux function 
p2 = 0;
if (xmax_top ~= xmin_top)
    p2 = 1 / (2 * (xmax_top - xmin_top));
end

== matlab function Model_TranslationEngine64/PostProcess/PostProcess/Soft Clipper/SoftClipper/translation1 ==
  data: xmin_top output; ymax_tune input; xmin_tune input; xmax_top output; p2 output
  events: trigger input FUNCTION_CALL_EVENT
function [xmin_top,xmax_top, p2] = fcn(ymax_tune, xmin_tune)

% Translates Ymax and Xmin to Xmax and Xmin

xmin_top = xmin_tune.Value;
xmax_top = 2 * ymax_tune.Value - xmin_top;

% p2 remains 0 unless below condition is met
% p2 is later used in the gain redux function 
p2 = 0;
if (xmax_top ~= xmin_top)
    p2 = 1 / (2 * (xmax_top - xmin_top));
end

== matlab function Model_TranslationEngine64/ModelPreAmp/DecRate/Medusa5H1/MedusaHoligram/Medusa5H1 Part 3/On/Full-rate Mixer/Full-Rate Mixer with CAE & Fade Ramper/Fade Tuning/Backward Downmix Max/Trivial Translation ==
  data: TOP output; BackwardDownmixMax input
  events: trigger input FUNCTION_CALL_EVENT
function TOP  = fcn(BackwardDownmixMax)
%#codegen
% Checks if the parameter satisfies dimensionality requirements
if(numel(BackwardDownmixMax.Value) ~= 1)
   TranslateError('The parameter ''medusa_backward_downmix_max'' must be single dimensional.'); 
end

% Checks if the parameter value follows bound requirements
if((BackwardDownmixMax.Value < 0) || (BackwardDownmixMax.Value > 1))
   TranslateError('The value of ''medusa_backward_downmix_max'' must be between 0 and 1.'); 
end

TOP = BackwardDownmixMax.Value;

end

== matlab function Model_TranslationEngine64/ModelPreAmp/DecRate/Medusa5H1/MedusaHoligram/Medusa5H1 Part 3/On/Full-rate Mixer/Full-Rate Mixer with CAE & Fade Ramper/Fade Tuning/Backward Downmix Threshold/Trivial Translation ==
  data: TOP output; BackwardDownmixThreshold input
  events: trigger input FUNCTION_CALL_EVENT
function TOP  = fcn(BackwardDownmixThreshold)
%#codegen
% Checks if the parameter satisfies dimensionality requirements
if(numel(BackwardDownmixThreshold.Value) ~= 1)
   TranslateError('The parameter ''medusa_backward_downmix_threshold'' must be single dimensional.'); 
end

% Checks if the parameter value follows bound requirements
if((BackwardDownmixThreshold.Value < 0) || (BackwardDownmixThreshold.Value > 1))
   TranslateError('The value of ''medusa_backward_downmix_threshold'' must be between 0 and 1.'); 
end

TOP = BackwardDownmixThreshold.Value;

end

== matlab function Model_TranslationEngine64/ModelPreAmp/DecRate/Medusa5H1/MedusaHoligram/Medusa5H1 Part 3/On/Full-rate Mixer/Full-Rate Mixer with CAE & Fade Ramper/Fade Tuning/Downmix Weights CS/Trivial Translation ==
  data: TOP output size=[MedusaFRMConfig.CS_out MedusaFRMConfig.CS_in]; downmix_wts_CS input; MedusaFRMConfig parameter; TOP_CAE output size=[MedusaFRMConfig.CS_out MedusaFRMConfig.NumTailComp.CS]
  events: trigger input FUNCTION_CALL_EVENT
function [TOP,TOP_CAE]  = fcn(downmix_wts_CS, MedusaFRMConfig)
%#codegen
numCSIn = MedusaFRMConfig.CS_in;
NumCAEWeights = MedusaFRMConfig.NumTailComp.CS;

NumRows = MedusaFRMConfig.CS_out;
NumColumns = numCSIn + NumCAEWeights;
if(~ MedusaFRMConfig.includeCAE)
    NumColumns = numCSIn;
end

% Checks if the parameter satisfies dimensionality requirements
if(downmix_wts_CS.Size(1) ~= NumRows || downmix_wts_CS.Size(2) ~= NumColumns)
    TranslateError('The parameter ''medusa_frm_downmix_cs'' must be a matrix consisting of %d rows and %d columns.', NumRows, NumColumns);
end

% Checks if the parameter values follow bound requirements
checkValues = (downmix_wts_CS.Value < 0);
if(sum(sum(checkValues)))          % Results in 0 if all values in the matrix respect the bound requirements
    TranslateError('The weights in ''medusa_frm_downmix_CS'' must be greater than or equal to 0.');
end

% Assigning the parameter values to respective tuneTOPS
TOP = downmix_wts_CS.Value(:, 1:numCSIn);
if(~ MedusaFRMConfig.includeCAE)
    TOP_CAE = zeros(NumRows, NumCAEWeights);
else
    TOP_CAE = downmix_wts_CS.Value(:, numCSIn+1:end);
end

end
